simulink model "NES1"  (R2019a)
settings: Solver=VariableStepAuto  StartTime=0.0  StopTime=10.0  RelTol=1e-3
InitFcn:
  | init
values from neighbouring files (symbols this model uses):
  c = params.c    [S2dot.m]    (also in cdisp.m; importdata.m = 100; ode45_code.m = 0.01)
  c_ij = [c1,c2,c3,c4]    [C_ij.m]    (also in C_ij1.m = double(c_ij); Main.m = C_ij2_coef(c_2dot); Vafaei.m = C_ij2_coef(c_2dot))
  cdot = Cdot_coef(c_2dot)    [Main.m]    (also in Vafaei.m)
  k = params.k    [S2dot.m]    (also in cdisp.m; importdata.m = 20000; main_QuestionE.m = 50000; ode45_code.m = 5)
  M = double(M)    [Resultant.m]
  m = params.m    [S2dot.m]    (also in importdata.m = 0.005; main_QuestionE.m = 527.1; ode45_code.m = 1)
  N = double(N)    [Resultant.m]
  Phi_i_star = double(Phi_i_star1)    [cdisp.m]
undefined symbols (not defined in the file or in its folder): c_ij2
settings Model: Creator=NegarPajooh  LastModifiedBy=NegarPajooh

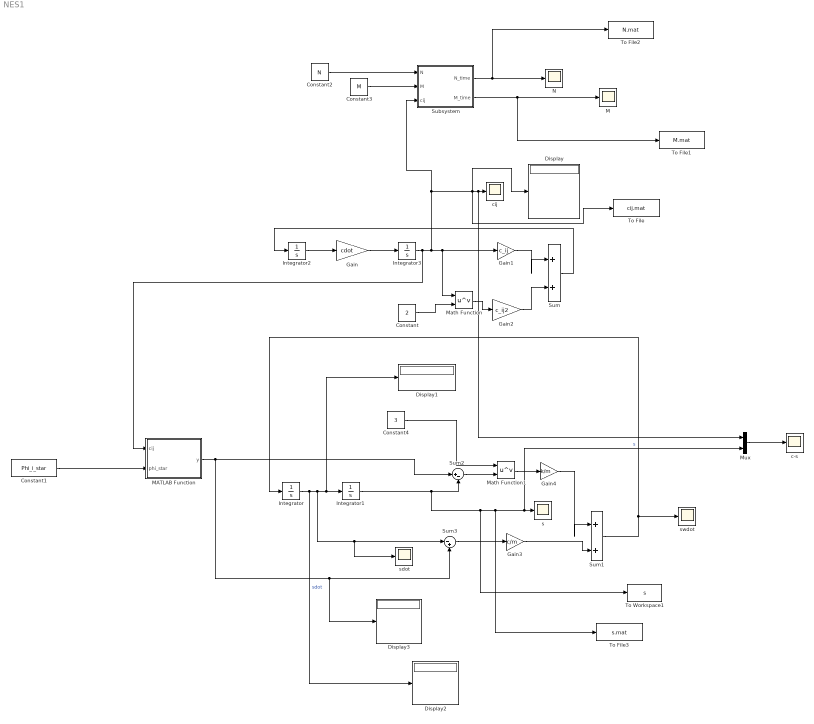
== system NES1 ==
  Constant : Constant  Value=2
  Constant1 : Constant  Value=Phi_i_star
  Constant2 : Constant  Value=N
  Constant3 : Constant  Value=M
  Constant4 : Constant  Value=3
  Display{,1..3} (4 alike) : Display
  Gain : Gain  Gain=cdot
  Gain1 : Gain  Gain=c_ij
  Gain2 : Gain  Gain=c_ij2
  Gain3 : Gain  Gain=c/m
  Gain4 : Gain  Gain=k/m
  Integrator{,1..3} (4 alike) : Integrator
  M : Scope
  MATLAB Function : MATLAB Function  TreatAsAtomicUnit=on
  Math Function : Math  Operator=pow  SaturateOnIntegerOverflow=on
  Math Function1 : Math  Operator=pow  SaturateOnIntegerOverflow=on
  Mux : Mux  Inputs=2
  N : Scope
  Subsystem : Subsystem
  Sum : Sum  Inputs=|++
  Sum1 : Sum  Inputs=|++
  Sum2 : Sum  Inputs=|+-
  Sum3 : Sum  Inputs=|-+
  To File : ToFile  Filename=cij.mat  MatrixName=cij
  To File1 : ToFile  Filename=M.mat  MatrixName=M
  To File2 : ToFile  Filename=N.mat  MatrixName=N
  To File3 : ToFile  Filename=s.mat  MatrixName=s  SaveFormat=Timeseries
  To Workspace1 : ToWorkspace  VariableName=s  SaveFormat=Structure With Time  SampleTime=-1
  c-s : Scope
  cij : Scope
  s : Scope
  sdot : Scope
  swdot : Scope
  wires:
  Integrator2/1 -> Gain/1
  Gain/1 -> Integrator3/1
  Constant/1 -> Math Function/2
  Math Function/1 -> Gain2/1
  Gain1/1 -> Sum/1
  Gain2/1 -> Sum/2
  Sum/1 -> Integrator2/1
  Integrator1/1 -> To Workspace1/1, To File3/1, Mux/2, s/1, Sum2/2  "s"
  MATLAB Function/1(y) -> Sum2/1, Display3/1, Sum3/2
  Sum1/1 -> swdot/1, Integrator/1
  Gain4/1 -> Sum1/1
  Sum3/1 -> Gain3/1
  Constant4/1 -> Math Function1/1
  Integrator/1 -> Display2/1, sdot/1, Sum3/1, Display1/1, Integrator1/1  "sdot"
  Sum2/1 -> Math Function1/2
  Math Function1/1 -> Gain4/1
  Gain3/1 -> Sum1/2
  Constant1/1 -> MATLAB Function/2(phi_star)
  Mux/1 -> c-s/1
  Subsystem/1("N_time ") -> To File2/1, N/1
  Subsystem/2("M_time ") -> To File1/1, M/1
  Constant3/1 -> Subsystem/2(M)
  Constant2/1 -> Subsystem/1(N)
  Integrator3/1 -> MATLAB Function/1(cij), Subsystem/3(cij), To File/1, Display/1, Mux/1, cij/1, Math Function/1, Gain1/1

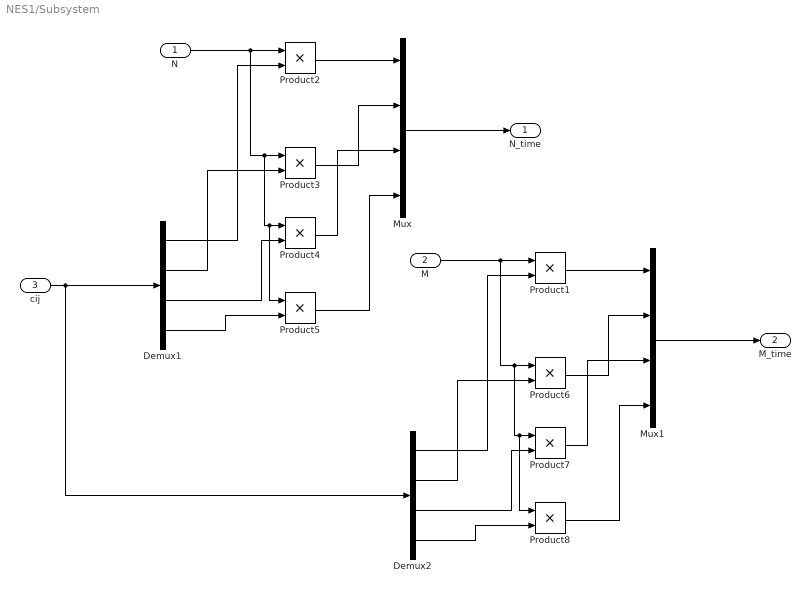
== system NES1/Subsystem ==
  N : Inport
  M : Inport  Port=2
  cij : Inport  Port=3
  Demux1 : Demux
  Demux2 : Demux
  Mux : Mux
  Mux1 : Mux
  Product{1..8} (8 alike) : Product
  "N_time " : Outport
  "M_time " : Outport  Port=2
  wires:
  Demux1/1 -> Product2/2
  Demux1/2 -> Product3/2
  Demux1/3 -> Product4/2
  Demux1/4 -> Product5/2
  N/1 -> Product5/1, Product4/1, Product3/1, Product2/1
  Product2/1 -> Mux/1
  Product3/1 -> Mux/2
  Product4/1 -> Mux/3
  Product5/1 -> Mux/4
  Mux/1 -> "N_time "/1
  Mux1/1 -> "M_time "/1
  Product8/1 -> Mux1/4
  Product7/1 -> Mux1/3
  Product6/1 -> Mux1/2
  Product1/1 -> Mux1/1
  M/1 -> Product1/1, Product6/1, Product7/1, Product8/1
  Demux2/4 -> Product8/2
  Demux2/3 -> Product7/2
  Demux2/2 -> Product6/2
  Demux2/1 -> Product1/2
  cij/1 -> Demux2/1, Demux1/1

== matlab function NES1/MATLAB Function ==
  data: cij input; y output; phi_star input
function y = fcn(cij,phi_star)
y1 = phi_star.*cij;
y =sum(y1);
end
